simulink model "MECH473Simp"  (R2017a)
settings: Solver=VariableStepAuto  StartTime=0.0  StopTime=100  RelTol=1e-3
values from neighbouring files (symbols this model uses):
  JM = 0.00026; sim('Mech473Simp'); plot(t,omega)    [boobies.m]
settings Model: Creator=ni_daly  LastModifiedBy=al_per

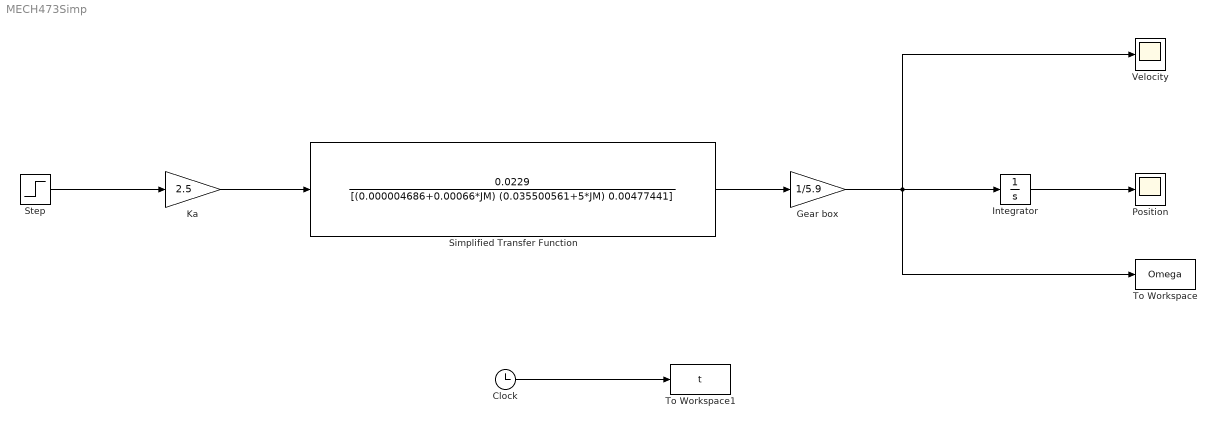
== system MECH473Simp ==
  Clock : Clock
  Gear box : Gain  Gain=1/5.9
  Integrator : Integrator
  Ka : Gain  Gain=2.5
  Position : Scope
  Simplified Transfer Function : TransferFcn  Numerator=[0.0229]  Denominator=[(0.000004686+0.00066*JM) (0.035500561+5*JM) 0.00477441]
  Step : Step  SampleTime=0
  To Workspace : ToWorkspace  VariableName=Omega  SampleTime=-1
  To Workspace1 : ToWorkspace  VariableName=t  SampleTime=-1
  Velocity : Scope
  wires:
  Clock/1 -> To Workspace1/1
  Simplified Transfer Function/1 -> Gear box/1
  Integrator/1 -> Position/1
  Step/1 -> Ka/1
  Ka/1 -> Simplified Transfer Function/1
  Gear box/1 -> To Workspace/1, Integrator/1, Velocity/1
